simulink model "CommandeVitesse"  (R2023a)
settings: Solver=VariableStepAuto  StartTime=0.0  StopTime=.2  FixedStep=0.0001  MaxStep=0.0001  RelTol=1e-3
undefined symbols (not defined in the file): f, J, Kc, Ke, L, R
settings Model: Creator=xpess  LastModifiedBy=xpess

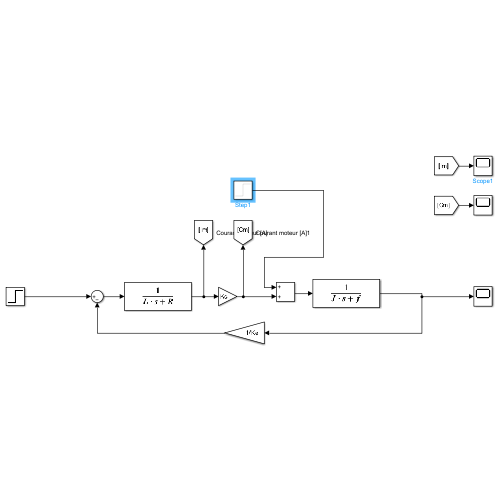
[thumbnail: Simulink's stored preview of the top-level diagram]
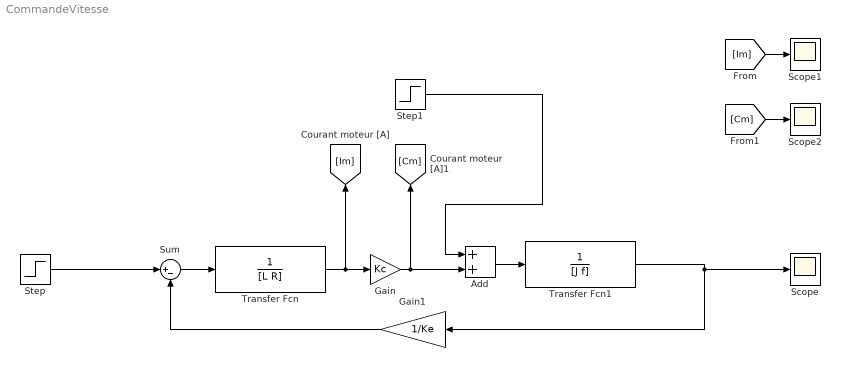
== system CommandeVitesse ==
  Add : Sum
  Gain : Gain  Gain=Kc
  Gain1 : Gain  Gain=1/Ke
  Scope : Scope
  Scope1 : Scope
  Scope2 : Scope
  Step : Step  Time=0  After=10  SampleTime=0
  Step1 : Step  Time=0  After=0  SampleTime=0
  Sum : Sum  Inputs=|+-
  Transfer Fcn : TransferFcn  Denominator=[L R]
  Transfer Fcn1 : TransferFcn  Denominator=[J f]
  wires:
  Transfer Fcn1/1 -> Scope/1, Gain1/1
  Gain/1 -> Add/2, [Cm]
  Gain1/1 -> Sum/2
  Step/1 -> Sum/1
  Transfer Fcn/1 -> Gain/1, [Im]
  [Im] -> Scope1/1
  Sum/1 -> Transfer Fcn/1
  [Cm] -> Scope2/1
  Add/1 -> Transfer Fcn1/1
  Step1/1 -> Add/1
